simulink library "MinSegLibrary_MinSegMega"  (R2015a)
settings: Solver=ode45  StartTime=0.0  StopTime=10.0  RelTol=1e-3
libraries: arduinolib x8, MinSegLibrary_M1V4 x1
settings Model: Creator=hurstj  LastModifiedBy=hurstj
settings DebuggingCC: UnderspecifiedInitializationDetection=Classic  MergeDetectMultiDrivingBlocksExec=none  SolverPrmCheckMsg=warning  StateNameClashWarn=warning

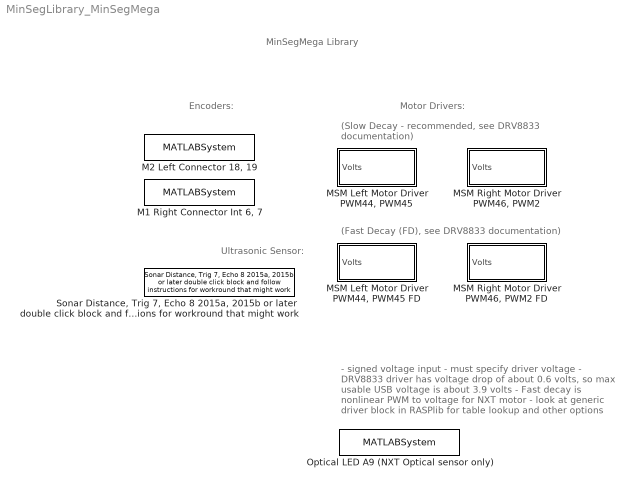
== system MinSegLibrary_MinSegMega ==
  note: (Slow Decay - recommended, see DRV8833 documentation)
  note: Motor Drivers:
  note: Ultrasonic Sensor:
  note: Encoders:
  note: MinSegMega Library
  note: (Fast Decay (FD), see DRV8833 documentation)
  note: - signed voltage input
      | - must specify driver voltage
      | - DRV8833 driver has voltage drop of about 0.6 volts, so max usable USB voltage is about 3.9 volts
      | - Fast decay is nonlinear PWM to voltage for NXT motor
      | - look at generic driver block in RASPlib for table lookup and other options
  "M1 Right Connector Int 6, 7" : MATLABSystem  System=Encoder_arduino  Encoder=2  PinA=6  PinB=7
      mask Type: Encoder_arduino
      mask Display:
      | disp('soEncoder');
      | port_label('output',1,'y');
  "M2 Left Connector 18, 19" : MATLABSystem  System=Encoder_arduino  Encoder=1  PinA=19  PinB=18
      mask Type: Encoder_arduino
      mask Display:
      | disp('soEncoder');
      | port_label('output',1,'y');
  "MSM Left Motor Driver PWM44, PWM45" : Subsystem  mask{Vsupply=3.9, PWMoffset=0}
      mask prompts: Vsupply "Driver Voltage"; PWMoffset "PWM offset (0-255)"
      mask help:
      | Specify driver supply voltage (3.9 for USB)
      | Specify the PWM offset (0-255)
      mask Display:
      | port_label('input',1,'Volts')
      | text(15,5,['Vsupply=' num2str(Vsupply)])
  "MSM Left Motor Driver PWM44, PWM45 FD" : Subsystem  mask{Vsupply=3.9, PWMoffset=0}
      mask prompts: Vsupply "Driver Voltage"; PWMoffset "PWM offset (0-255)"
      mask help:
      | Specify driver supply voltage (3.9 for USB)
      | Specify the PWM offset (0-255)
      mask Display:
      | port_label('input',1,'Volts')
      | text(15,5,['Vsupply=' num2str(Vsupply)])
  "MSM Right Motor Driver PWM46, PWM2 " : Subsystem  mask{Vsupply=3.9, PWMoffset=0}
      mask prompts: Vsupply "Driver Voltage"; PWMoffset "PWM offset (0-255)"
      mask help:
      | Specify driver supply voltage (3.9 for USB)
      | Specify the PWM offset (0-255)
      mask Display:
      | port_label('input',1,'Volts')
      | text(15,5,['Vsupply=' num2str(Vsupply)])
  "MSM Right Motor Driver PWM46, PWM2 FD" : Subsystem  mask{Vsupply=3.9, PWMoffset=0}
      mask prompts: Vsupply "Driver Voltage"; PWMoffset "PWM offset (0-255)"
      mask help:
      | Specify driver supply voltage (3.9 for USB)
      | Specify the PWM offset (0-255)
      mask Display:
      | port_label('input',1,'Volts')
      | text(15,5,['Vsupply=' num2str(Vsupply)])
  Optical LED A9 (NXT Optical sensor only) : MATLABSystem  System=soDAnalogWrite  Pin=9
      mask Type: soDAnalogWrite
      mask Display:
      | disp('Analog Digital Write');
      | port_label('input',1,'u');
  "Sonar Distance, Trig 7, Echo 8 2015a, 2015b or later double click block and follow instructions for workround that might work" : MinSegLibrary_M1V4/Sonar Distance, Trig 7, Echo 8 2015a, 2015b or later double click block and follow instructions for workround that might work  Sonar=1  TrigPin=7  EchoPin=8

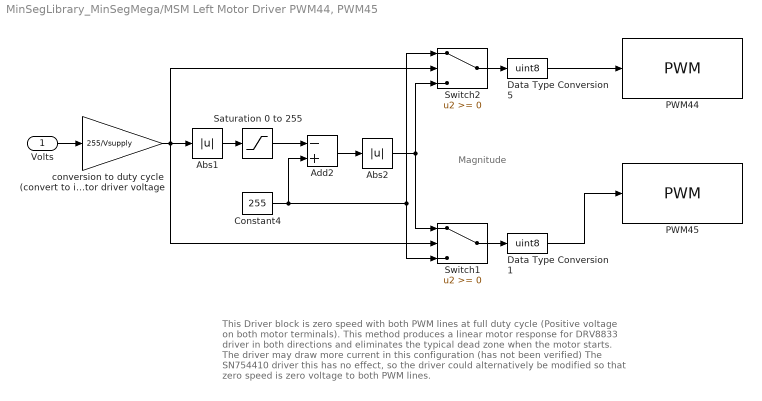
== system MinSegLibrary_MinSegMega/MSM Left Motor Driver PWM44, PWM45 ==
  note: Magnitude
  note: This Driver block is zero speed with both PWM lines at full duty cycle
      |  (Positive voltage on both motor terminals).
      | This method produces a linear motor response for DRV8833 driver
      |  in both directions and eliminates
      | the typical dead zone when the motor starts.
      | The driver may draw more current in this configuration (has not been verified)
      |
      | The SN754410 driver this has no effect, so the driver could alternatively
      | be modified so that zero speed is zero voltage to both PWM lines.
  Volts : Inport
  Abs1 : Abs
  Abs2 : Abs
  Add2 : Sum  Inputs=-+
  Constant4 : Constant  Value=255
  Data Type Conversion1 : DataTypeConversion  OutDataTypeStr=uint8
  Data Type Conversion5 : DataTypeConversion  OutDataTypeStr=uint8
  PWM44 : arduinolib/PWM  pinNumber=44  blockPlatform=arduino
  PWM45 : arduinolib/PWM  pinNumber=45  blockPlatform=arduino
  Saturation 0 to 255 : Saturate  UpperLimit=255  LowerLimit=0
  Switch1 : Switch
  Switch2 : Switch
  conversion to duty cycle (convert to int) denominator is motor driver voltage : Gain  Gain=255/Vsupply  OutDataTypeStr=int16
  wires:
  Data Type Conversion1/1 -> PWM45/1
  Data Type Conversion5/1 -> PWM44/1
  Switch1/1 -> Data Type Conversion1/1
  Switch2/1 -> Data Type Conversion5/1
  Abs2/1 -> Switch1/1, Switch2/3
  Add2/1 -> Abs2/1
  Constant4/1 -> Add2/2, Switch2/1, Switch1/3
  Abs1/1 -> Saturation 0 to 255/1
  Saturation 0 to 255/1 -> Add2/1
  conversion to duty cycle (convert to int) denominator is motor driver voltage/1 -> Switch1/2, Abs1/1, Switch2/2
  Volts/1 -> conversion to duty cycle (convert to int) denominator is motor driver voltage/1

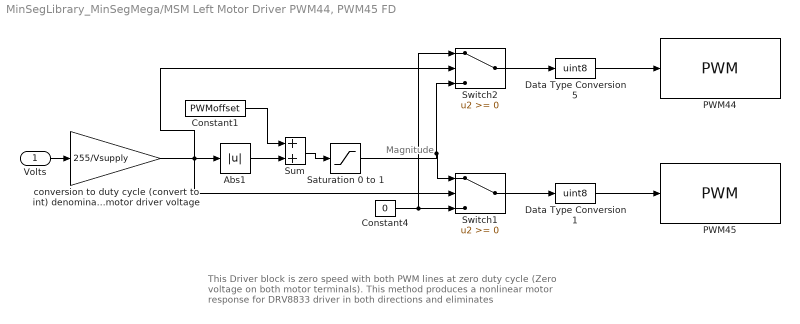
== system MinSegLibrary_MinSegMega/MSM Left Motor Driver PWM44, PWM45 FD ==
  note: Magnitude
  note: This Driver block is zero speed with both PWM lines at zero duty cycle
      |  (Zero voltage on both motor terminals).
      | This method produces a nonlinear motor response for DRV8833 driver
      |  in both directions and eliminates
  Volts : Inport
  Abs1 : Abs
  Constant1 : Constant  Value=PWMoffset
  Constant4 : Constant  Value=0
  Data Type Conversion1 : DataTypeConversion  OutDataTypeStr=uint8
  Data Type Conversion5 : DataTypeConversion  OutDataTypeStr=uint8
  PWM44 : arduinolib/PWM  pinNumber=44  blockPlatform=arduino
  PWM45 : arduinolib/PWM  pinNumber=45  blockPlatform=arduino
  Saturation 0 to 1 : Saturate  UpperLimit=255  LowerLimit=0
  Sum : Sum
  Switch1 : Switch
  Switch2 : Switch
  conversion to duty cycle (convert to int) denominator is motor driver voltage : Gain  Gain=255/Vsupply  OutDataTypeStr=int16
  wires:
  Constant1/1 -> Sum/1
  Sum/1 -> Saturation 0 to 1/1
  Abs1/1 -> Sum/2
  Data Type Conversion1/1 -> PWM45/1
  Data Type Conversion5/1 -> PWM44/1
  Switch1/1 -> Data Type Conversion1/1
  Switch2/1 -> Data Type Conversion5/1
  Saturation 0 to 1/1 -> Switch1/1, Switch2/3
  Constant4/1 -> Switch1/3, Switch2/1
  conversion to duty cycle (convert to int) denominator is motor driver voltage/1 -> Switch2/2, Abs1/1, Switch1/2
  Volts/1 -> conversion to duty cycle (convert to int) denominator is motor driver voltage/1

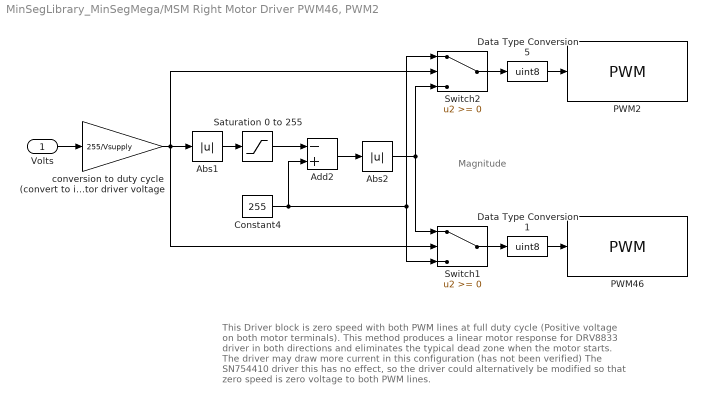
== system MinSegLibrary_MinSegMega/MSM Right Motor Driver PWM46, PWM2  ==
  note: Magnitude
  note: This Driver block is zero speed with both PWM lines at full duty cycle
      |  (Positive voltage on both motor terminals).
      | This method produces a linear motor response for DRV8833 driver
      |  in both directions and eliminates
      | the typical dead zone when the motor starts.
      | The driver may draw more current in this configuration (has not been verified)
      |
      | The SN754410 driver this has no effect, so the driver could alternatively
      | be modified so that zero speed is zero voltage to both PWM lines.
  Volts : Inport
  Abs1 : Abs
  Abs2 : Abs
  Add2 : Sum  Inputs=-+
  Constant4 : Constant  Value=255
  Data Type Conversion1 : DataTypeConversion  OutDataTypeStr=uint8
  Data Type Conversion5 : DataTypeConversion  OutDataTypeStr=uint8
  PWM2 : arduinolib/PWM  pinNumber=2  blockPlatform=arduino
  PWM46 : arduinolib/PWM  pinNumber=46  blockPlatform=arduino
  Saturation 0 to 255 : Saturate  UpperLimit=255  LowerLimit=0
  Switch1 : Switch
  Switch2 : Switch
  conversion to duty cycle (convert to int) denominator is motor driver voltage : Gain  Gain=255/Vsupply  OutDataTypeStr=int16
  wires:
  Data Type Conversion1/1 -> PWM46/1
  Data Type Conversion5/1 -> PWM2/1
  Switch1/1 -> Data Type Conversion1/1
  Switch2/1 -> Data Type Conversion5/1
  Abs2/1 -> Switch1/1, Switch2/3
  Add2/1 -> Abs2/1
  Constant4/1 -> Add2/2, Switch2/1, Switch1/3
  Abs1/1 -> Saturation 0 to 255/1
  Saturation 0 to 255/1 -> Add2/1
  conversion to duty cycle (convert to int) denominator is motor driver voltage/1 -> Switch1/2, Switch2/2, Abs1/1
  Volts/1 -> conversion to duty cycle (convert to int) denominator is motor driver voltage/1

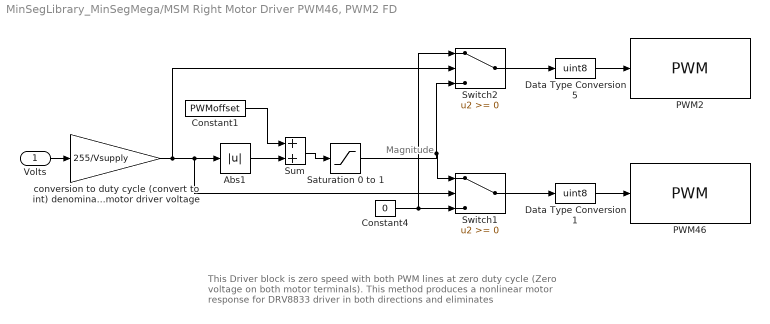
== system MinSegLibrary_MinSegMega/MSM Right Motor Driver PWM46, PWM2 FD ==
  note: Magnitude
  note: This Driver block is zero speed with both PWM lines at zero duty cycle
      |  (Zero voltage on both motor terminals).
      | This method produces a nonlinear motor response for DRV8833 driver
      |  in both directions and eliminates
  Volts : Inport
  Abs1 : Abs
  Constant1 : Constant  Value=PWMoffset
  Constant4 : Constant  Value=0
  Data Type Conversion1 : DataTypeConversion  OutDataTypeStr=uint8
  Data Type Conversion5 : DataTypeConversion  OutDataTypeStr=uint8
  PWM2 : arduinolib/PWM  pinNumber=2  blockPlatform=arduino
  PWM46 : arduinolib/PWM  pinNumber=46  blockPlatform=arduino
  Saturation 0 to 1 : Saturate  UpperLimit=255  LowerLimit=0
  Sum : Sum
  Switch1 : Switch
  Switch2 : Switch
  conversion to duty cycle (convert to int) denominator is motor driver voltage : Gain  Gain=255/Vsupply  OutDataTypeStr=int16
  wires:
  Constant1/1 -> Sum/1
  Sum/1 -> Saturation 0 to 1/1
  Abs1/1 -> Sum/2
  Data Type Conversion1/1 -> PWM46/1
  Data Type Conversion5/1 -> PWM2/1
  Switch1/1 -> Data Type Conversion1/1
  Switch2/1 -> Data Type Conversion5/1
  Saturation 0 to 1/1 -> Switch1/1, Switch2/3
  Constant4/1 -> Switch1/3, Switch2/1
  conversion to duty cycle (convert to int) denominator is motor driver voltage/1 -> Switch2/2, Abs1/1, Switch1/2
  Volts/1 -> conversion to duty cycle (convert to int) denominator is motor driver voltage/1
